simulink model "IMSpeedControl"  (R2022b)
settings: Solver=VariableStepAuto  StartTime=0.0  StopTime=55  RelTol=1e-3
values from neighbouring files (symbols this model uses):
  Bet = 0.068    [Induction_motor_parameters.m]
  isdn = 20.33    [Induction_motor_parameters.m]
  isqn = 2.12    [Induction_motor_parameters.m]
  J = [0 -1;1 0]    [Induction_motor_parameters.m]
  Jeq = 0.4    [Induction_motor_parameters.m]
  K = 0.009    [Induction_motor_parameters.m]
  Kip = Kpp/ Tip    (= 8.13922028395)    [Induction_motor_parameters.m]
  Kiw = 1.8    [Induction_motor_parameters.m]
  Kp = 5/0.001*Lks    (= 22.1269035533)    [Induction_motor_parameters.m]
  Kpp = 5/0.1*Lm    (= 2.74873096447)    [Induction_motor_parameters.m]
  Kpw = 1.1    [Induction_motor_parameters.m]
  Lks = Ls-Lm    (= 0.00442538071066)    [Induction_motor_parameters.m]
  Lks_ = [Lks 0;0 Lks]    [Induction_motor_parameters.m]
  Lm = Lm^2/Lr    (= 0.0549746192893)    [Induction_motor_parameters.m]
  Lm_ = [Lm 0;0 Lm]    [Induction_motor_parameters.m]
  np = 3    [Induction_motor_parameters.m]
  Rr = Rr*Lm^2/Lr^2    (= 0.162784405679)    [Induction_motor_parameters.m]
  Rr_ = [Rr 0;0 Rr]    [Induction_motor_parameters.m]
  Rs_ = [Rs 0;0 Rs]    [Induction_motor_parameters.m]
  Ti = Lks/Rks    (= 0.0109869713133)    [Induction_motor_parameters.m]
  wb = 104.61    [Induction_motor_parameters.m]
undefined symbols (not defined in the file or in its folder): Inv_Clarke, Inv_Park, Park, sigbuilder_block
settings Model: Creator=Utente  LastModifiedBy=Davvy
settings SolverCC: AlgebraicLoopSolver=TrustRegion
settings DataIOCC: ReturnWorkspaceOutputs=off
settings DebuggingCC: UnconnectedInputMsg=warning  UnconnectedOutputMsg=warning  UnconnectedLineMsg=warning  SFMachineParentedDataDiag=warning  ArithmeticOperatorsInVariantConditions=warning
settings ModelReferenceCC: EnableRefExpFcnMdlSchedulingChecks=on
settings SFSimCC: SimUseLocalCustomCode=off  CustomCodeUndefinedFunction=UseInterfaceOnly
settings RTWCC: RTWUseLocalCustomCode=off  DLArmComputeVersion=19.05
settings CodeAppCC: StateflowObjectComments=on

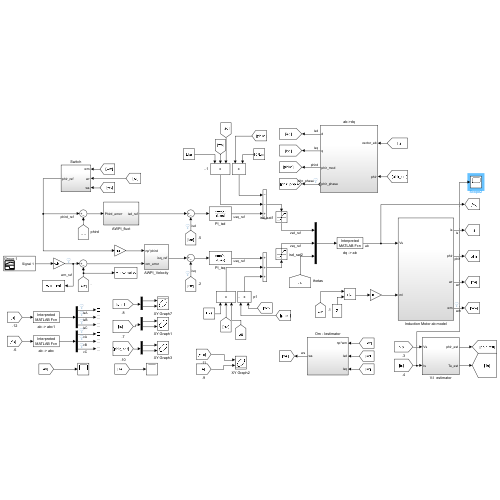
[thumbnail: Simulink's stored preview of the top-level diagram]
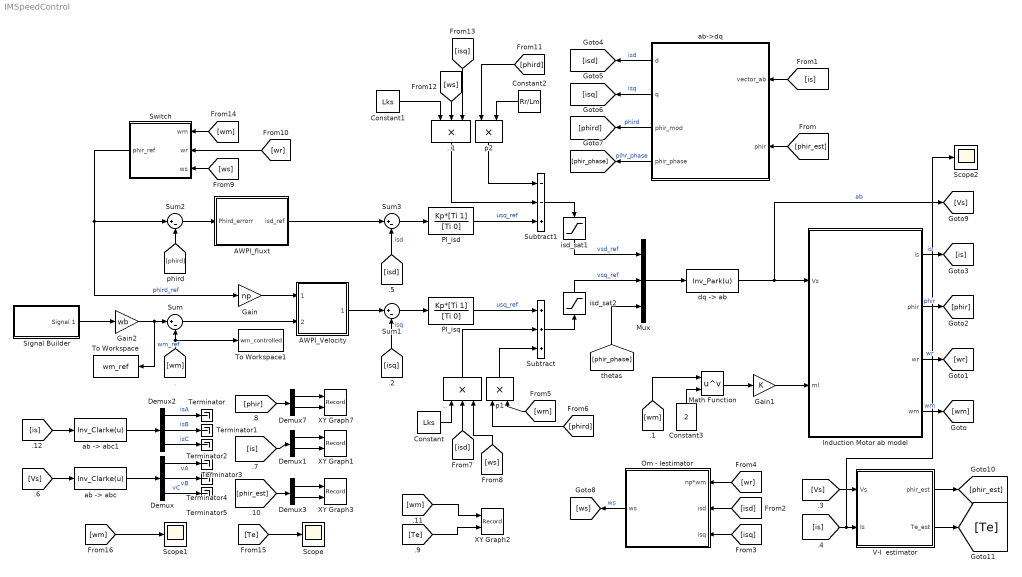
== system IMSpeedControl ==
  .. : Product  Inputs=***
  ..1 : Product  Inputs=***
  AWPI_Velocity : Subsystem
  AWPI_fluxt : Subsystem
  Constant : Constant  Value=Lks
  Constant1 : Constant  Value=Lks
  Constant2 : Constant  Value=Rr/Lm
  Constant3 : Constant  Value=2
  Demux : Demux  Outputs=3
  Demux1 : Demux  Outputs=2
  Demux2 : Demux  Outputs=3
  Demux3 : Demux  Outputs=2
  Demux7 : Demux  Outputs=2
  Gain : Gain  Gain=np
  Gain1 : Gain  Gain=K
  Gain2 : Gain  Gain=wb
  Induction Motor ab model : Subsystem
  Math Function : Math  Operator=pow  SignedPower=on
  Mux : Mux  Inputs=3
  Om - Iestimator : Subsystem
  PI_isd : TransferFcn  Numerator=Kp*[Ti 1]  Denominator=[Ti 0]
  PI_isq : TransferFcn  Numerator=Kp*[Ti 1]  Denominator=[Ti 0]
  Scope : Scope
  Scope1 : Scope
  Scope2 : Scope
  Signal Builder : Subsystem  Tag=STV Subsys  LoadFcn=sigbuilder_block('load');  StartFcn=sigbuilder_block('start');  StopFcn=sigbuilder_block('stop');  ClipboardFcn=sigbuilder_block('clipboard');  mask(Sigbuilder block){tuvar=[0:10]}
      mask help: Simulink:masks:SigbuilderBlock_MD
      mask init:
      | if ~strcmp(get_param(bdroot(gcbh),'SimulationStatus'),'stopped') tuvar = sigbuilder_block('maskInit'); end
      settings: CopyFcn=sigbuilder_block('copy');  DeleteFcn=sigbuilder_block('delete');  ModelCloseFcn=sigbuilder_block('modelClose');  PreSaveFcn=sigbuilder_block('preSave');  PauseFcn=sigbuilder_block('pause');  ContinueFcn=sigbuilder_block('continue');  NameChangeFcn=sigbuilder_block('namechange');  OpenFcn=sigbuilder_block('open',[6 30 1012.5 447.75 ]);  CloseFcn=sigbuilder_block('close');
      mask Display: plot(0, 0, 100, 100,[2, 2, 32, 32, 2], [68, 8, 8, 68, 68],[32, 2], [38, 38], [32, 19, 2],[53, 60, 44], [32, 17, 17, 2],[16, 16, 31, 31]);txt = getActiveGroup(gcbh);text(2, 100, txt,'verticalAlignment', 'top');
  Subtract : Sum  Inputs=+++
  Subtract1 : Sum  Inputs=--+
  Sum{,1..3} (4 alike) : Sum  Inputs=|+-
  Switch : Subsystem
  Terminator{,1..5} (6 alike) : Terminator
  To Workspace : ToWorkspace  VariableName=wm_ref  SaveFormat=Timeseries  SampleTime=-1
  To Workspace1 : ToWorkspace  VariableName=wm_controlled  SaveFormat=Timeseries  SampleTime=-1
  V-I  estimator : Subsystem
  XY Graph1 : Record  FileSettingsInternal="{\"entries\":[{\"content\":{\"excelSettings\":{\"content\":{},\"type\":\"Streamout.ExcelSettings\"}},\"type\":\"Streamout.FileSettingStorage\",\"uuid\":\"d3ca43fa-2eb8-43c5-9975-2b22932f402f\"}],\"packageUris\":[\"http://schema.mathworks.com/mf0/streamout_blocks/R2020a\"],\"version\":\"1.0\"}"  Layout=[1 1]  SignalsInternal="{\"entries\":[{\"content\":{\"signals\":[{\"content\":{\"blockPath\":[\"IMSpeedControl/XY Graph1\"],\"channel\":[],\"dimensions\":[1],\"domain\":\"IMSpeedControl/XY Graph1\",\"lineColor\":\"#a2142f\",\"plots\":[1],\"port\":1,\"sid\":[\"\"],\"signalID\":2589,\"signalName\":\"Demux1:1\"},\"type\":\"RecordBlkView.Signal\",\"uuid\":\"02de77b0-35d0-4548-bb27-b905c8801d44\"},{\"content\":{\"blockPath\":[\"IMSpeedControl/XY Graph1\"],\"channel\":[],\"dimensions\":[1],\"domain\":\"IMSpeedControl/XY Graph1\",\"lineColor\":\"#139fff\",\"plots\":[1],\"port\":2,\"sid\":[\"\"],\"signalID\":2593,\"signalName\":\"Demux1:2\"},\"type\":\"RecordBlkView.Signal\",\"uuid\":\"53935ca3-2f54-4a23-9646-f53dd009e972\"}]},\"type\":\"RecordBlkView.InputSignals\",\"uuid\":\"47193afe-2425-4409-be18-3384f797a584\"}],\"packageUris\":[\"http://schema.mathworks.com/mf0/streamout_blocks/R2020a\"],\"version\":\"1.0\"}"  VisualizationBindings="{\"xyplotplugin\":{\"info\":[{\"series\":[{\"bindingParametersList\":[{\"parameter\":\"X-Axis\",\"signalID\":2589,\"signalName\":\"Demux1:1\"},{\"parameter\":\"Y-Axis\",\"signalID\":2593,\"signalName\":\"Demux1:2\"}],\"seriesID\":41022}],\"subplotID\":1}]}}"  CompatibilityTag=XY  st=-1
  XY Graph2 : Record  FileSettingsInternal="{\"entries\":[{\"content\":{\"excelSettings\":{\"content\":{},\"type\":\"Streamout.ExcelSettings\"}},\"type\":\"Streamout.FileSettingStorage\",\"uuid\":\"a333dde8-44ef-479c-a614-b682ced7709c\"}],\"packageUris\":[\"http://schema.mathworks.com/mf0/streamout_blocks/R2020a\"],\"version\":\"1.0\"}"  Layout=[1 1]  SignalsInternal="{\"entries\":[{\"content\":{\"signals\":[{\"content\":{\"blockPath\":[\"IMSpeedControl/XY Graph2\"],\"channel\":[],\"dimensions\":[1],\"domain\":\"IMSpeedControl/XY Graph2\",\"lineColor\":\"#a2142f\",\"plots\":[1],\"port\":1,\"sid\":[\"\"],\"signalID\":2597,\"signalName\":\".11\"},\"type\":\"RecordBlkView.Signal\",\"uuid\":\"f7e30db1-32b0-4ca4-8bfd-82b278195b5f\"},{\"content\":{\"blockPath\":[\"IMSpeedControl/XY Graph2\"],\"channel\":[],\"dimensions\":[1],\"domain\":\"IMSpeedControl/XY Graph2\",\"lineColor\":\"#139fff\",\"plots\":[1],\"port\":2,\"sid\":[\"\"],\"signalID\":2601,\"signalName\":\".9\"},\"type\":\"RecordBlkView.Signal\",\"uuid\":\"c26b9c31-f389-46e3-b070-48b4825ac3b8\"}]},\"type\":\"RecordBlkView.InputSignals\",\"uuid\":\"892b814f-ea27-4dea-9e30-1f6eece8a5fc\"}],\"packageUris\":[\"http://schema.mathworks.com/mf0/streamout_blocks/R2020a\"],\"version\":\"1.0\"}"  VisualizationBindings="{\"xyplotplugin\":{\"info\":[{\"series\":[{\"bindingParametersList\":[{\"parameter\":\"X-Axis\",\"signalID\":2597,\"signalName\":\".11\"},{\"parameter\":\"Y-Axis\",\"signalID\":2601,\"signalName\":\".9\"}],\"seriesID\":14013}],\"subplotID\":1}]}}"  CompatibilityTag=XY  st=-1
  XY Graph3 : Record  FileSettingsInternal="{\"entries\":[{\"content\":{\"excelSettings\":{\"content\":{},\"type\":\"Streamout.ExcelSettings\"}},\"type\":\"Streamout.FileSettingStorage\",\"uuid\":\"8872b38d-c9ea-4a8e-ae80-a4eae1dd000b\"}],\"packageUris\":[\"http://schema.mathworks.com/mf0/streamout_blocks/R2020a\"],\"version\":\"1.0\"}"  Layout=[1 1]  SignalsInternal="{\"entries\":[{\"content\":{\"signals\":[{\"content\":{\"blockPath\":[\"IMSpeedControl/XY Graph3\"],\"channel\":[],\"dimensions\":[1],\"domain\":\"IMSpeedControl/XY Graph3\",\"lineColor\":\"#a2142f\",\"plots\":[1],\"port\":1,\"sid\":[\"\"],\"signalID\":2605,\"signalName\":\"Demux3:1\"},\"type\":\"RecordBlkView.Signal\",\"uuid\":\"8f683524-bb5c-486f-9abb-78ec64469034\"},{\"content\":{\"blockPath\":[\"IMSpeedControl/XY Graph3\"],\"channel\":[],\"dimensions\":[1],\"domain\":\"IMSpeedControl/XY Graph3\",\"lineColor\":\"#139fff\",\"plots\":[1],\"port\":2,\"sid\":[\"\"],\"signalID\":2609,\"signalName\":\"Demux3:2\"},\"type\":\"RecordBlkView.Signal\",\"uuid\":\"ce7d3715-b402-496e-9cf6-d9fdbd852528\"}]},\"type\":\"RecordBlkView.InputSignals\",\"uuid\":\"2dbcf389-952d-43f2-8df1-56cbfee3bb29\"}],\"packageUris\":[\"http://schema.mathworks.com/mf0/streamout_blocks/R2020a\"],\"version\":\"1.0\"}"  VisualizationBindings="{\"xyplotplugin\":{\"info\":[{\"series\":[{\"bindingParametersList\":[{\"parameter\":\"X-Axis\",\"signalID\":2605,\"signalName\":\"Demux3:1\"},{\"parameter\":\"Y-Axis\",\"signalID\":2609,\"signalName\":\"Demux3:2\"}],\"seriesID\":20617}],\"subplotID\":1}]}}"  CompatibilityTag=XY  st=-1
  XY Graph7 : Record  FileSettingsInternal="{\"entries\":[{\"content\":{\"excelSettings\":{\"content\":{},\"type\":\"Streamout.ExcelSettings\"}},\"type\":\"Streamout.FileSettingStorage\",\"uuid\":\"0bf42496-7210-4f3b-99f3-3b3a1dd7ec81\"}],\"packageUris\":[\"http://schema.mathworks.com/mf0/streamout_blocks/R2020a\"],\"version\":\"1.0\"}"  Layout=[1 1]  SignalsInternal="{\"entries\":[{\"content\":{\"signals\":[{\"content\":{\"blockPath\":[\"IMSpeedControl/XY Graph7\"],\"channel\":[],\"dimensions\":[1],\"domain\":\"IMSpeedControl/XY Graph7\",\"lineColor\":\"#a2142f\",\"plots\":[1],\"port\":1,\"sid\":[\"\"],\"signalID\":2613,\"signalName\":\"Demux7:1\"},\"type\":\"RecordBlkView.Signal\",\"uuid\":\"cdc689f2-e2ee-4a3d-8cbf-3711711c7aba\"},{\"content\":{\"blockPath\":[\"IMSpeedControl/XY Graph7\"],\"channel\":[],\"dimensions\":[1],\"domain\":\"IMSpeedControl/XY Graph7\",\"lineColor\":\"#139fff\",\"plots\":[1],\"port\":2,\"sid\":[\"\"],\"signalID\":2617,\"signalName\":\"Demux7:2\"},\"type\":\"RecordBlkView.Signal\",\"uuid\":\"bf97ebbf-5e9a-4653-b8b6-6523d9603def\"}]},\"type\":\"RecordBlkView.InputSignals\",\"uuid\":\"f683bfae-dbd4-4a57-97ca-43081def8fa8\"}],\"packageUris\":[\"http://schema.mathworks.com/mf0/streamout_blocks/R2020a\"],\"version\":\"1.0\"}"  VisualizationBindings="{\"xyplotplugin\":{\"info\":[{\"series\":[{\"bindingParametersList\":[{\"parameter\":\"X-Axis\",\"signalID\":2613,\"signalName\":\"Demux7:1\"},{\"parameter\":\"Y-Axis\",\"signalID\":2617,\"signalName\":\"Demux7:2\"}],\"seriesID\":21423}],\"subplotID\":1}]}}"  CompatibilityTag=XY  st=-1
  "ab -> abc" : MATLABFcn  MATLABFcn=Inv_Clarke(u)  OutputSignalType=real
  "ab -> abc1" : MATLABFcn  MATLABFcn=Inv_Clarke(u)  OutputSignalType=real
  ab->dq : Subsystem
  "dq -> ab" : MATLABFcn  MATLABFcn=Inv_Park(u)  OutputDimensions=2  OutputSignalType=real
  isd_sat1 : Saturate  UpperLimit=380  LowerLimit=-380
  isd_sat2 : Saturate  UpperLimit=380  LowerLimit=-380
  p1 : Product  Inputs=**
  p2 : Product  Inputs=**
  wires:
  "dq -> ab"/1 -> [Vs], Induction Motor ab model/1(Vs)  "ab"
  Mux/1 -> "dq -> ab"/1
  Induction Motor ab model/4(wm) -> [wm]  "wm"
  Induction Motor ab model/3(wr) -> [wr]  "wr"
  Induction Motor ab model/2(phir) -> [phir]  "phir"
  Induction Motor ab model/1(is) -> [is]  "is"
  [phir_est] -> ab->dq/2(phir)
  [is] -> ab->dq/1(vector_ab)
  ab->dq/1(d) -> [isd]  "isd"
  ab->dq/2(q) -> [isq]  "isq"
  ab->dq/3(phir_mod) -> [phird]  "phird"
  ab->dq/4(phir_phase) -> [phir_phase]  "pihr_phase"
  [wm] -> To Workspace1/1, Sum/2
  Sum/1 -> AWPI_Velocity/2(om_error)
  [phird] -> Sum2/2
  Gain/1 -> AWPI_Velocity/1(np*phird)
  [isq] -> Sum1/2  "isq"
  Sum1/1 -> PI_isq/1
  PI_isq/1 -> Subtract/1  "usq_ref"
  [isd] -> Om - Iestimator/2(isd)
  [wr] -> Om - Iestimator/1(np*wm)
  [isq] -> Om - Iestimator/3(isq)
  [wm] -> p1/2
  [phird] -> p1/1
  p1/1 -> Subtract/3
  [isd] -> ../2
  [ws] -> ../3
  Constant/1 -> ../1
  ../1 -> Subtract/2
  Subtract/1 -> isd_sat2/1
  Constant1/1 -> ..1/1
  [ws] -> ..1/2
  Subtract1/1 -> isd_sat1/1
  Switch/1(phir_ref) -> Gain/1, Sum2/1  "phird_ref"
  [phird] -> p2/1
  Sum2/1 -> AWPI_fluxt/1(Phird_errorr)
  Sum3/1 -> PI_isd/1
  [isq] -> ..1/3
  p2/1 -> Subtract1/1
  Constant2/1 -> p2/2
  ..1/1 -> Subtract1/2
  PI_isd/1 -> Subtract1/3  "usq_ref"
  [isd] -> Sum3/2  "isd"
  Gain1/1 -> Induction Motor ab model/2(ml)
  [ws] -> Switch/3(ws)
  [wr] -> Switch/2(wr)
  [wm] -> Switch/1(wm)
  [phir_phase] -> Mux/3
  [Vs] -> V-I  estimator/1(Vs)
  [is] -> Scope2/1, V-I  estimator/2(Is)
  V-I  estimator/1(phir_est) -> [phir_est]
  isd_sat2/1 -> Mux/2  "vsq_ref"
  isd_sat1/1 -> Mux/1  "vsd_ref"
  AWPI_fluxt/1(isd_ref) -> Sum3/1
  AWPI_Velocity/1(isq_ref) -> Sum1/1
  Math Function/1 -> Gain1/1
  [wm] -> Math Function/1
  Constant3/1 -> Math Function/2
  "ab -> abc"/1 -> Demux/1
  Demux/1 -> Terminator3/1  "vA"
  Demux/2 -> Terminator4/1  "vB"
  Demux/3 -> Terminator5/1  "vC"
  [Vs] -> "ab -> abc"/1
  Demux1/1 -> XY Graph1/1
  Demux1/2 -> XY Graph1/2
  Signal Builder/1(Signal 1) -> Gain2/1
  Gain2/1 -> To Workspace/1, Sum/1  "wm_ref"
  Om - Iestimator/1(ws) -> [ws]  "ws"
  [is] -> Demux1/1
  Demux7/1 -> XY Graph7/1
  Demux7/2 -> XY Graph7/2
  [phir] -> Demux7/1
  [wm] -> XY Graph2/1
  [Te] -> XY Graph2/2
  Demux3/1 -> XY Graph3/1
  [phir_est] -> Demux3/1
  Demux3/2 -> XY Graph3/2
  V-I  estimator/2(Te_est) -> [Te]
  Demux2/2 -> Terminator1/1  "isB"
  Demux2/3 -> Terminator2/1  "isC"
  Demux2/1 -> Terminator/1  "isA"
  [is] -> "ab -> abc1"/1
  "ab -> abc1"/1 -> Demux2/1
  [Te] -> Scope/1
  [wm] -> Scope1/1

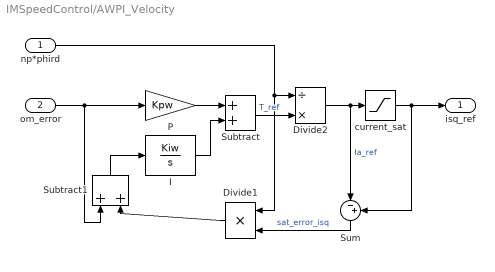
== system IMSpeedControl/AWPI_Velocity ==
  np*phird : Inport
  om_error : Inport  Port=2
  Divide1 : Product  Inputs=**
  Divide2 : Product  Inputs=/*
  I : TransferFcn  Numerator=Kiw  Denominator=[1 0]
  P : Gain  Gain=Kpw
  Subtract : Sum
  Subtract1 : Sum
  Sum : Sum  Inputs=|-+
  current_sat : Saturate  UpperLimit=isqn  LowerLimit=-isqn
  isq_ref : Outport
  wires:
  P/1 -> Subtract/1
  om_error/1 -> Subtract1/1, P/1
  Divide2/1 -> Sum/1, current_sat/1  "Ia_ref"
  Subtract/1 -> Divide2/2  "T_ref"
  np*phird/1 -> Divide1/1, Divide2/1
  current_sat/1 -> Sum/2, isq_ref/1
  Subtract1/1 -> I/1
  Sum/1 -> Divide1/2  "sat_error_isq"
  I/1 -> Subtract/2
  Divide1/1 -> Subtract1/2

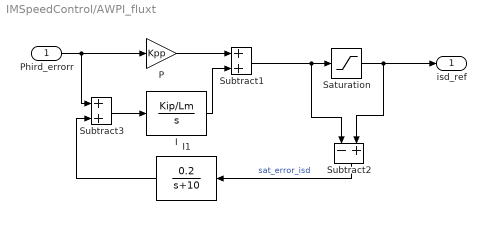
== system IMSpeedControl/AWPI_fluxt ==
  Phird_errorr : Inport
  I : TransferFcn  Numerator=Kip/Lm  Denominator=[1 0]
  I1 : TransferFcn  Numerator=0.2  Denominator=[1 10]
  P : Gain  Gain=Kpp
  Saturation : Saturate  UpperLimit=isdn  LowerLimit=-isdn
  Subtract1 : Sum
  Subtract2 : Sum  Inputs=-+
  Subtract3 : Sum
  isd_ref : Outport
  wires:
  Subtract1/1 -> Subtract2/1, Saturation/1
  Phird_errorr/1 -> Subtract3/1, P/1
  I/1 -> Subtract1/2
  P/1 -> Subtract1/1
  Saturation/1 -> Subtract2/2, isd_ref/1
  Subtract3/1 -> I/1
  Subtract2/1 -> I1/1  "sat_error_isd"
  I1/1 -> Subtract3/2

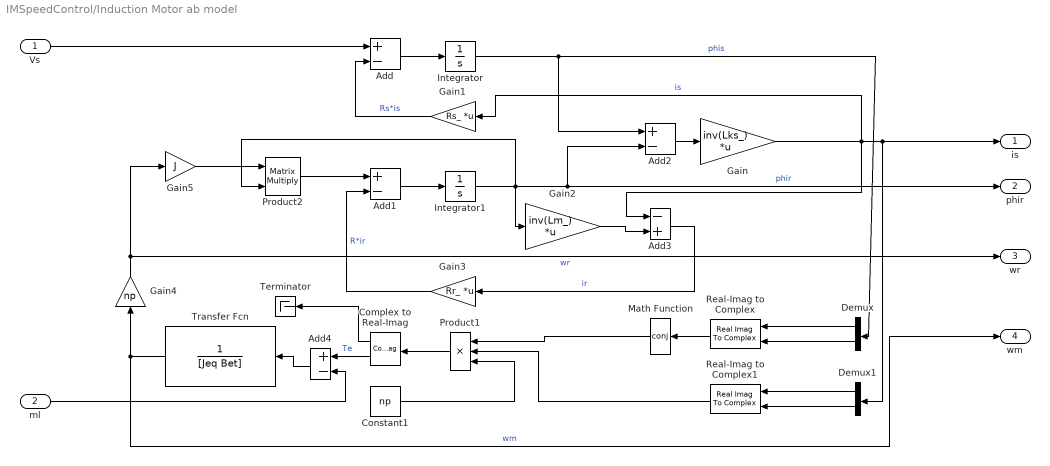
== system IMSpeedControl/Induction Motor ab model ==
  Vs : Inport
  ml : Inport  Port=2
  Add : Sum  Inputs=+-
  Add1 : Sum  Inputs=+-  InputSameDT=on
  Add2 : Sum  Inputs=+-
  Add3 : Sum  Inputs=-+
  Add4 : Sum  Inputs=+-
  Complex to Real-Imag : ComplexToRealImag
  Constant1 : Constant  Value=np
  Demux : Demux  Outputs=2
  Demux1 : Demux  Outputs=2
  Gain : Gain  Gain=inv(Lks_)  Multiplication=Matrix(K*u)
  Gain1 : Gain  Gain=Rs_  Multiplication=Matrix(K*u)
  Gain2 : Gain  Gain=inv(Lm_)  Multiplication=Matrix(K*u)
  Gain3 : Gain  Gain=Rr_  Multiplication=Matrix(K*u)
  Gain4 : Gain  Gain=np
  Gain5 : Gain  Gain=J
  Integrator : Integrator
  Integrator1 : Integrator
  Math Function : Math  Operator=conj  SignedPower=on
  Product1 : Product  Inputs=3
  Product2 : Product  Multiplication=Matrix(*)
  Real-Imag to Complex : RealImagToComplex
  Real-Imag to Complex1 : RealImagToComplex
  Terminator : Terminator
  Transfer Fcn : TransferFcn  Denominator=[Jeq Bet]
  is : Outport
  phir : Outport  Port=2
  wr : Outport  Port=3
  wm : Outport  Port=4
  wires:
  Add1/1 -> Integrator1/1
  Gain1/1 -> Add/2  "Rs*is"
  Add/1 -> Integrator/1
  ml/1 -> Add4/2
  Constant1/1 -> Product1/3
  Add4/1 -> Transfer Fcn/1
  Complex to Real-Imag/2 -> Add4/1  "Te"
  Transfer Fcn/1 -> wm/1, Gain4/1  "wm"
  Math Function/1 -> Product1/1
  Vs/1 -> Add/1
  Product1/1 -> Complex to Real-Imag/1
  Integrator/1 -> Demux/1, Add2/1  "phis"
  Product2/1 -> Add1/1
  Integrator1/1 -> Product2/2, Add2/2, phir/1, Gain2/1  "phir"
  Add3/1 -> Gain3/1  "ir"
  Gain4/1 -> wr/1, Gain5/1  "wr"
  Gain/1 -> Gain1/1, Demux1/1, is/1, Add3/1  "is"
  Gain2/1 -> Add3/2
  Add2/1 -> Gain/1
  Gain3/1 -> Add1/2  "R*ir"
  Demux/2 -> Real-Imag to Complex/2
  Demux/1 -> Real-Imag to Complex/1
  Real-Imag to Complex/1 -> Math Function/1
  Demux1/2 -> Real-Imag to Complex1/2
  Demux1/1 -> Real-Imag to Complex1/1
  Real-Imag to Complex1/1 -> Product1/2
  Gain5/1 -> Product2/1
  Complex to Real-Imag/1 -> Terminator/1

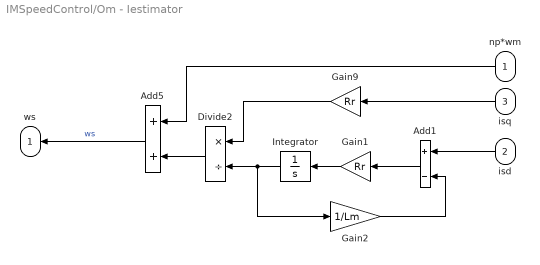
== system IMSpeedControl/Om - Iestimator ==
  np*wm : Inport
  isd : Inport  Port=2
  isq : Inport  Port=3
  Add1 : Sum  Inputs=+-
  Add5 : Sum
  Divide2 : Product  Inputs=*/
  Gain1 : Gain  Gain=Rr
  Gain2 : Gain  Gain=1/Lm
  Gain9 : Gain  Gain=Rr
  Integrator : Integrator  InitialCondition=1.1
  ws : Outport
  wires:
  isq/1 -> Gain9/1
  Divide2/1 -> Add5/2
  Gain9/1 -> Divide2/1
  Add5/1 -> ws/1  "ws"
  np*wm/1 -> Add5/1
  Gain1/1 -> Integrator/1
  Integrator/1 -> Gain2/1, Divide2/2
  Add1/1 -> Gain1/1
  Gain2/1 -> Add1/2
  isd/1 -> Add1/1

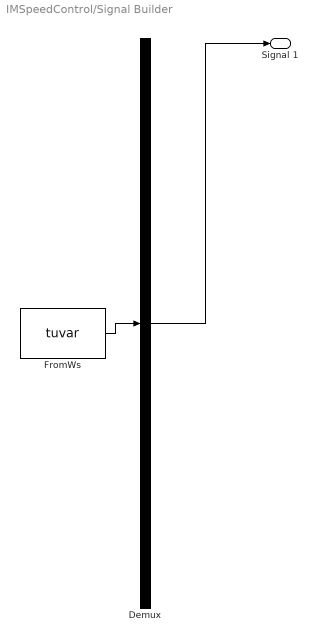
== system IMSpeedControl/Signal Builder ==
  Demux : Demux  Tag=STV Demux  Outputs=1
      settings: DisplayOption=none
  FromWs : FromWorkspace  Tag=STV FromWs  VariableName=tuvar
      SigBuilderData=|
      | common.afterFinalStr = 'Extrapolate'
      | common.sampleTime = 0
      | dataSet.timeRange = [0 70]
      | dataSet.name = 'Group 1'
      | sbobj.Groups.Name = 'Group 1'
      | sbobj.Groups.Signals.Name = 'Signal 1'
      | sbobj.Groups.Signals.XData = [0 20 30 40 50 55 70]
      | sbobj.Groups.Signals.YData = [0 0.1 0.1 0.2 0.2 0.2 0.2]
      | sbobj.Groups.TimeRange = [0 70]
  Signal 1 : Outport  Tag=STV Outport
  wires:
  Demux/1 -> Signal 1/1
  FromWs/1 -> Demux/1

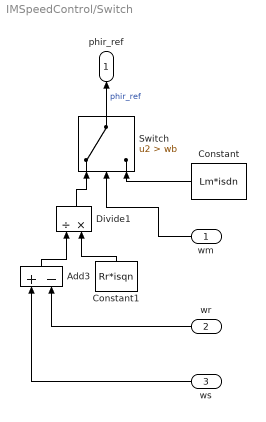
== system IMSpeedControl/Switch ==
  wm : Inport
  wr : Inport  Port=2
  ws : Inport  Port=3
  Add3 : Sum  Inputs=+-
  Constant : Constant  Value=Lm*isdn
  Constant1 : Constant  Value=Rr*isqn
  Divide1 : Product  Inputs=/*
  Switch : Switch  Criteria=u2 > Threshold  Threshold=wb  SaturateOnIntegerOverflow=off  InputSameDT=off
  phir_ref : Outport
  wires:
  wm/1 -> Switch/2
  ws/1 -> Add3/1
  Add3/1 -> Divide1/1
  Constant1/1 -> Divide1/2
  Divide1/1 -> Switch/1
  Constant/1 -> Switch/3
  Switch/1 -> phir_ref/1  "phir_ref"
  wr/1 -> Add3/2

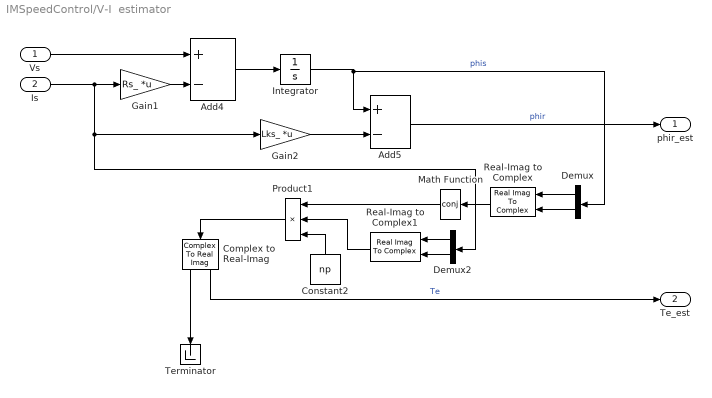
== system IMSpeedControl/V-I  estimator ==
  Vs : Inport
  Is : Inport  Port=2
  Add4 : Sum  Inputs=+-
  Add5 : Sum  Inputs=+-
  Complex to Real-Imag : ComplexToRealImag
  Constant2 : Constant  Value=np
  Demux : Demux  Outputs=2
  Demux2 : Demux  Outputs=2
  Gain1 : Gain  Gain=Rs_  Multiplication=Matrix(K*u)
  Gain2 : Gain  Gain=Lks_  Multiplication=Matrix(K*u)
  Integrator : Integrator
  Math Function : Math  Operator=conj  SignedPower=on
  Product1 : Product  Inputs=3
  Real-Imag to Complex : RealImagToComplex
  Real-Imag to Complex1 : RealImagToComplex
  Terminator : Terminator
  phir_est : Outport
  Te_est : Outport  Port=2
  wires:
  Add4/1 -> Integrator/1
  Add5/1 -> phir_est/1  "phir"
  Vs/1 -> Add4/1
  Gain1/1 -> Add4/2
  Real-Imag to Complex1/1 -> Product1/2
  Demux/1 -> Real-Imag to Complex/1
  Demux/2 -> Real-Imag to Complex/2
  Is/1 -> Demux2/1, Gain2/1, Gain1/1
  Constant2/1 -> Product1/3
  Integrator/1 -> Add5/1, Demux/1  "phis"
  Math Function/1 -> Product1/1
  Real-Imag to Complex/1 -> Math Function/1
  Complex to Real-Imag/2 -> Te_est/1  "Te"
  Demux2/2 -> Real-Imag to Complex1/2
  Demux2/1 -> Real-Imag to Complex1/1
  Product1/1 -> Complex to Real-Imag/1
  Gain2/1 -> Add5/2
  Complex to Real-Imag/1 -> Terminator/1

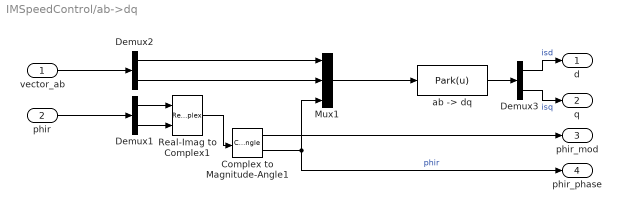
== system IMSpeedControl/ab->dq ==
  vector_ab : Inport
  phir : Inport  Port=2
  Complex to Magnitude-Angle1 : ComplexToMagnitudeAngle
  Demux1 : Demux  Outputs=2
  Demux2 : Demux  Outputs=2
  Demux3 : Demux  Outputs=2
  Mux1 : Mux  Inputs=3
  Real-Imag to Complex1 : RealImagToComplex
  "ab -> dq" : MATLABFcn  MATLABFcn=Park(u)  OutputDimensions=2
  d : Outport
  q : Outport  Port=2
  phir_mod : Outport  Port=3
  phir_phase : Outport  Port=4
  wires:
  vector_ab/1 -> Demux2/1
  Demux3/1 -> d/1  "isd"
  phir/1 -> Demux1/1
  Complex to Magnitude-Angle1/2 -> Mux1/3, phir_phase/1  "phir"
  Real-Imag to Complex1/1 -> Complex to Magnitude-Angle1/1
  Demux1/2 -> Real-Imag to Complex1/2
  Demux1/1 -> Real-Imag to Complex1/1
  Demux2/1 -> Mux1/1
  Mux1/1 -> "ab -> dq"/1
  Demux2/2 -> Mux1/2
  Demux3/2 -> q/1  "isq"
  "ab -> dq"/1 -> Demux3/1
  Complex to Magnitude-Angle1/1 -> phir_mod/1
